simulink model "APID_RLS"  (R2021b)
settings: Solver=ode5  StartTime=0.0  StopTime=5000  FixedStep=0.2  RelTol=1e-3  EnableMultiTasking=on
undefined symbols (not defined in the file or in its folder): Disturb, setSimFuncRLS
settings Model: SimulationMode=accelerator  Creator=issme  LastModifiedBy=ismt
settings SolverCC: AlgebraicLoopSolver=TrustRegion
settings DataIOCC: SaveFormat=Array  SignalLoggingSaveFormat=ModelDataLogs  ReturnWorkspaceOutputs=off  OutputSaveName=yout_RLS
settings OptimizationCC: ExpressionDepthLimit=2147483647  InitFltsAndDblsToZero=on  LifeSpan=inf
settings DebuggingCC: UnderspecifiedInitializationDetection=Classic  MergeDetectMultiDrivingBlocksExec=none  SolverPrmCheckMsg=warning  FcnCallInpInsideContextMsg=warning  StateNameClashWarn=warning  SFUnexpectedBacktrackingDiag=warning  SFNoUnconditionalDefaultTransitionDiag=warning  SFExecutionAtInitializationDiag=none  SFMachineParentedDataDiag=warning  ArithmeticOperatorsInVariantConditions=warning
settings HardwareCC: ProdBitPerPointer=32  ProdBitPerSizeT=32  ProdBitPerPtrDiffT=32  ProdLargestAtomicFloat=None  ProdIntDivRoundTo=Undefined  ProdEndianess=Unspecified  ProdWordSize=32  ProdHWDeviceType=32-bit Generic
settings ModelReferenceCC: PropagateSignalLabelsOutOfModel=off
settings CodeAppCC: StateflowObjectComments=on
settings GRTTargetCC: TargetLangStandard=C89/C90 (ANSI)  CombineOutputUpdateFcns=off  GRTInterface=on
settings ConfigComp: CovMetricSettings=dw  CovSaveCumulativeToWorkspaceVar=on  CovSaveSingleToWorkspaceVar=on

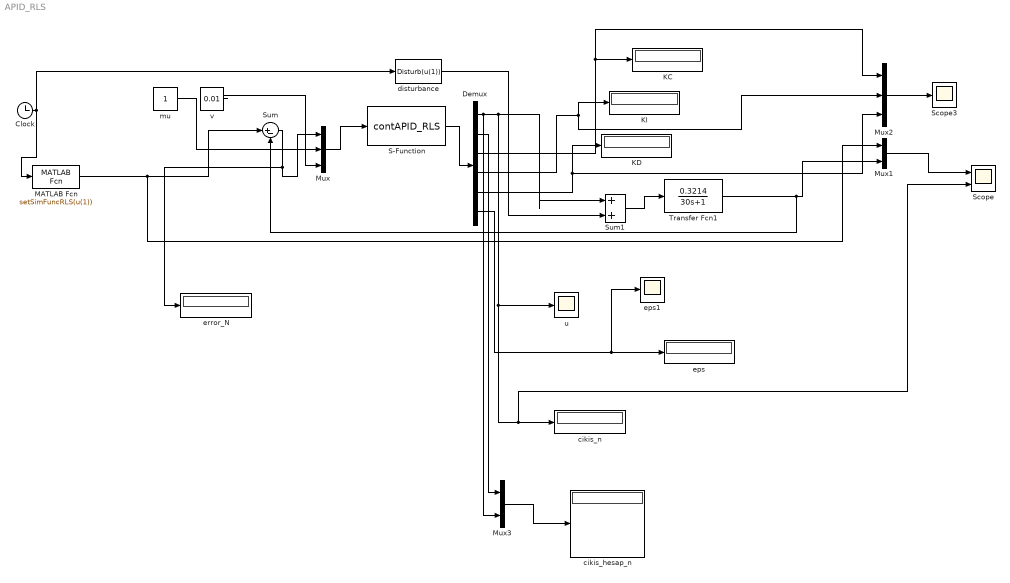
== system APID_RLS ==
  Clock : Clock
  Demux : Demux  Outputs=6
  KC : Display
  KD : Display
  KI : Display
  MATLAB Fcn : MATLABFcn  MATLABFcn=setSimFuncRLS(u(1))
  Mux : Mux  Inputs=3
  Mux1 : Mux  Inputs=2
  Mux2 : Mux  Inputs=3
  Mux3 : Mux  Inputs=2
  S-Function : S-Function  FunctionName=contAPID_RLS  SFunctionDeploymentMode=off  EnableBusSupport=off
  Scope : Scope  NumInputPorts=2
  Scope3 : Scope
  Sum : Sum  Inputs=|+-
  Sum1 : Sum  Inputs=|++
  Transfer Fcn1 : TransferFcn  Numerator=0.3214  Denominator=[30 1]
  cikis_hesap_n : Display
  cikis_n : Display
  disturbance : MATLABFcn  MATLABFcn=Disturb(u(1))
  eps : Display
  eps1 : Scope
  error_N : Display
  mu : Constant
  u : Scope
  v : Constant  Value=0.01
  wires:
  MATLAB Fcn/1 -> Mux1/1, Sum/1
  Sum/1 -> error_N/1, Mux/1
  mu/1 -> Mux/2
  v/1 -> Mux/3
  Mux/1 -> S-Function/1
  S-Function/1 -> Demux/1
  Clock/1 -> MATLAB Fcn/1, disturbance/1
  Sum1/1 -> Transfer Fcn1/1
  Mux1/1 -> Scope/1
  Mux2/1 -> Scope3/1
  Mux3/1 -> cikis_hesap_n/1
  Demux/1 -> Scope/2, cikis_n/1, u/1, Sum1/1, Mux3/2
  disturbance/1 -> Sum1/2
  Demux/2 -> Mux3/1
  Demux/3 -> Mux2/1, KC/1
  Demux/4 -> KI/1, Mux2/2
  Demux/5 -> KD/1, Mux2/3
  Demux/6 -> eps1/1, eps/1
  Transfer Fcn1/1 -> Sum/2, Mux1/2
